simulink model "fec_ber_hw_V2"  (R2020b)
settings: Solver=FixedStepDiscrete  StartTime=0.0  StopTime=T  RelTol=1e-3
values from neighbouring files (symbols this model uses):
  aximm_awgn_reset = 0    [setup.m]
  aximm_bit_count_reset = 0    [setup.m]
  aximm_bits = n_blocks * k    (= 80)    [setup.m]
  aximm_ctrl_word_dec = 0    [setup.m]
  aximm_ctrl_word_enc = 0    [setup.m]
  aximm_enable = 1    [setup.m]
  aximm_length = k * n_blocks    (= 80)    [setup.m]
  aximm_length_dec = n    (= 160)    [setup.m]
  aximm_length_enc = k    (= 80)    [setup.m]
  aximm_llr_mag_reset = 0    [setup.m]
  aximm_llr_scale = (1/noise_var) * llr_scale    (= 1000)    [setup.m]
  aximm_load_dec = 1    [setup.m]
  aximm_load_enc = 1    [setup.m]
  aximm_noise_std = sqrt(noise_var)    [setup.m]
  aximm_reset = 0    [setup.m]
  d = sqrt(-2*log([0:1/4095:1]))    [setup.m]
  fs = 160e6    (= 160000000)    [setup.m]
  generator_polynomial = '''z^13 + z^12 + z^11 + z^8 + 1'''    [setup.m]
  llr_scale = 7.75/7.75    (= 1)    [setup.m]
libraries: simulink x931, hdlsllib x419, commseqgen3 x52, dspsigops x22, commblkcod2 x3, lib_rfsoc_fec x2
(part 47 of 47)

== stateflow chart fec_ber_hw_V2/Encoder Ctrl/Chart ==
  settings: executeAtInitialization=1
  state INIT
    % Local
    count = fi(0,0,32,0);
    n = fi(0,0,32,0);
    loaded_n = fi(0,0,32,0);
    loaded_ctrl = fi(0,0,32,0);
    %
    % DATA Stream
    m_axis_tvalid = false;
    m_axis_tdata = fi(0,0,32,0);
    %
    % CTRL Stream
    m_axis_ctrl_tdata = fi(0,0,32,0);
    m_axis_ctrl_tlast = false;
    m_axis_ctrl_tvalid = false;
    %
    % STATUS Stream
    s_axis_status_tready = false;
  state IDLE
    % Local
    %
    % DATA Stream
    m_axis_tvalid(:) = false;
    m_axis_tdata(:) = 0;
    %
    % CTRL Stream
    m_axis_ctrl_tdata = fi(0,0,32,0);
    m_axis_ctrl_tlast = false;
    m_axis_ctrl_tvalid = false;
    %
    % STATUS Stream
    s_axis_status_tready = false;
  state LOAD_NVALID
    % Local
    loaded_n(:) = block_length;
    loaded_ctrl(:) = ctrl_word;
    %
    % DATA Stream
    m_axis_tvalid(:) = false;
    m_axis_tdata(:) = 0;
    %
    % CTRL Stream
    m_axis_ctrl_tdata(:) = 0;
    m_axis_ctrl_tlast(:) = false;
    m_axis_ctrl_tvalid(:) = false;
    %
    % STATUS Stream
    s_axis_status_tready(:) = true;
  state LOAD_VALID
    % Local
    count(:) = count + 1;
    loaded_n(:) = block_length;
    loaded_ctrl(:) = ctrl_word;
    %
    % DATA Stream
    m_axis_tvalid(:) = true;
    m_axis_tdata(:) = s_axis_tdata;
    %
    % CTRL Stream
    m_axis_ctrl_tdata(:) = 0;
    m_axis_ctrl_tlast(:) = false;
    m_axis_ctrl_tvalid(:) = false;
    %
    % STATUS Stream
    s_axis_status_tready(:) = true;
  state COUNT_DIN
    % Local
    count(:) = count + 1;
    %
    % DATA Stream
    m_axis_tvalid(:) = true;
    m_axis_tdata(:) = s_axis_tdata;       % Complete a full block
    %
    % CTRL Stream
    m_axis_ctrl_tdata(:) = 0;
    m_axis_ctrl_tlast(:) = false;
    m_axis_ctrl_tvalid(:) = false;
    %
    % STATUS Stream
    s_axis_status_tready(:) = true;
  state CTRL
    % Local
    count(:) = count + 1;
    n(:) = loaded_n;
    %
    % DATA Stream
    m_axis_tvalid(:) = true;
    m_axis_tdata(:) = s_axis_tdata;
    %
    % CTRL Stream
    m_axis_ctrl_tdata(:) = loaded_ctrl;
    m_axis_ctrl_tlast(:) = true;
    m_axis_ctrl_tvalid(:) = true;
    %
    % STATUS Stream
    s_axis_status_tready(:) = true;
  state WAITING
    % Local
    %
    % DATA Stream
    m_axis_tvalid(:) = false;
    m_axis_tdata(:) = s_axis_tdata;
    %
    % CTRL Stream
    m_axis_ctrl_tdata(:) = 0;
    m_axis_ctrl_tlast(:) = false;
    m_axis_ctrl_tvalid(:) = false;
    %
    % STATUS Stream
    s_axis_status_tready(:) = true;
  LOAD_VALID -> IDLE [order 3] : [count >= n && s_axis_tvalid == 0]{count(:) = 0}
  (default) -> INIT
  LOAD_NVALID -> COUNT_DIN [order 2] : [s_axis_tvalid == 1 && count > 0]
  LOAD_VALID -> CTRL [order 2] : [count >= n && s_axis_tvalid == 1]{count(:) = 0}
  IDLE -> LOAD_NVALID [order 1] : [load == 1]
  INIT -> IDLE
  LOAD_VALID -> COUNT_DIN [order 1] : [count < n]
  CTRL -> LOAD_VALID [order 1] : [load == 1 && s_axis_tvalid == 1]
  COUNT_DIN -> LOAD_NVALID [order 5] : [load == 1 && s_axis_tvalid == 0]
  LOAD_NVALID -> CTRL [order 1] : [s_axis_tvalid == 1 && count ==0]
  COUNT_DIN -> IDLE [order 3] : [count >= n && s_axis_tvalid == 0]{count(:) = 0}
  IDLE -> CTRL [order 2] : [s_axis_tvalid == 1 && count ==0]
  COUNT_DIN -> LOAD_VALID [order 2] : [load == 1 && s_axis_tvalid == 1]
  COUNT_DIN -> WAITING [order 4] : [load == 0 && s_axis_tvalid == 0]
  CTRL -> COUNT_DIN [order 2] : [s_axis_tvalid == 1]
  COUNT_DIN -> CTRL [order 1] : [count >= n && s_axis_tvalid == 1]{count(:) = 0}
  WAITING -> COUNT_DIN : [s_axis_tvalid == 1]
  CTRL -> WAITING [order 3] : [s_axis_tvalid == 0]
  data: m_axis_ctrl_tvalid output; ctrl_word input; count local; m_axis_ctrl_tdata output; m_axis_ctrl_tlast output; m_axis_tvalid output; block_length input; load input; s_axis_tvalid input; s_axis_status_tready output; n local; loaded_ctrl local; loaded_n local; state output Enum: stateType; s_axis_tdata input; m_axis_tdata output

== matlab function fec_ber_hw_V2/Soft Demodulation/SSR Soft Demodulation Lane 2/Soft Demodulation 10/symmetric_saturation ==
  data: u input; y output
function y = symmetric_saturation(u)
    if u > 7.75
        y = fi(7.75, 1, 6, 2);
    elseif u < -7.75
        y = fi(-7.75, 1, 6, 2);
    else
        y = fi(u, 1, 6, 2);
    end

== matlab function fec_ber_hw_V2/Soft Demodulation/SSR Soft Demodulation Lane 2/Soft Demodulation 11/symmetric_saturation ==
  data: u input; y output
function y = symmetric_saturation(u)
    if u > 7.75
        y = fi(7.75, 1, 6, 2);
    elseif u < -7.75
        y = fi(-7.75, 1, 6, 2);
    else
        y = fi(u, 1, 6, 2);
    end

== matlab function fec_ber_hw_V2/Soft Demodulation/SSR Soft Demodulation Lane 2/Soft Demodulation 12/symmetric_saturation ==
  data: u input; y output
function y = symmetric_saturation(u)
    if u > 7.75
        y = fi(7.75, 1, 6, 2);
    elseif u < -7.75
        y = fi(-7.75, 1, 6, 2);
    else
        y = fi(u, 1, 6, 2);
    end

== matlab function fec_ber_hw_V2/Soft Demodulation/SSR Soft Demodulation Lane 2/Soft Demodulation 13/symmetric_saturation ==
  data: u input; y output
function y = symmetric_saturation(u)
    if u > 7.75
        y = fi(7.75, 1, 6, 2);
    elseif u < -7.75
        y = fi(-7.75, 1, 6, 2);
    else
        y = fi(u, 1, 6, 2);
    end

== matlab function fec_ber_hw_V2/Soft Demodulation/SSR Soft Demodulation Lane 2/Soft Demodulation 14/symmetric_saturation ==
  data: u input; y output
function y = symmetric_saturation(u)
    if u > 7.75
        y = fi(7.75, 1, 6, 2);
    elseif u < -7.75
        y = fi(-7.75, 1, 6, 2);
    else
        y = fi(u, 1, 6, 2);
    end

== matlab function fec_ber_hw_V2/Soft Demodulation/SSR Soft Demodulation Lane 2/Soft Demodulation 15/symmetric_saturation ==
  data: u input; y output
function y = symmetric_saturation(u)
    if u > 7.75
        y = fi(7.75, 1, 6, 2);
    elseif u < -7.75
        y = fi(-7.75, 1, 6, 2);
    else
        y = fi(u, 1, 6, 2);
    end

== matlab function fec_ber_hw_V2/Soft Demodulation/SSR Soft Demodulation Lane 3/Soft Demodulation 1/symmetric_saturation ==
  data: u input; y output
function y = symmetric_saturation(u)
    if u > 7.75
        y = fi(7.75, 1, 6, 2);
    elseif u < -7.75
        y = fi(-7.75, 1, 6, 2);
    else
        y = fi(u, 1, 6, 2);
    end

== matlab function fec_ber_hw_V2/Soft Demodulation/SSR Soft Demodulation Lane 3/Soft Demodulation 2/symmetric_saturation ==
  data: u input; y output
function y = symmetric_saturation(u)
    if u > 7.75
        y = fi(7.75, 1, 6, 2);
    elseif u < -7.75
        y = fi(-7.75, 1, 6, 2);
    else
        y = fi(u, 1, 6, 2);
    end

== matlab function fec_ber_hw_V2/Soft Demodulation/SSR Soft Demodulation Lane 3/Soft Demodulation 3/symmetric_saturation ==
  data: u input; y output
function y = symmetric_saturation(u)
    if u > 7.75
        y = fi(7.75, 1, 6, 2);
    elseif u < -7.75
        y = fi(-7.75, 1, 6, 2);
    else
        y = fi(u, 1, 6, 2);
    end

== matlab function fec_ber_hw_V2/Soft Demodulation/SSR Soft Demodulation Lane 3/Soft Demodulation 4/symmetric_saturation ==
  data: u input; y output
function y = symmetric_saturation(u)
    if u > 7.75
        y = fi(7.75, 1, 6, 2);
    elseif u < -7.75
        y = fi(-7.75, 1, 6, 2);
    else
        y = fi(u, 1, 6, 2);
    end

== matlab function fec_ber_hw_V2/Soft Demodulation/SSR Soft Demodulation Lane 3/Soft Demodulation 5/symmetric_saturation ==
  data: u input; y output
function y = symmetric_saturation(u)
    if u > 7.75
        y = fi(7.75, 1, 6, 2);
    elseif u < -7.75
        y = fi(-7.75, 1, 6, 2);
    else
        y = fi(u, 1, 6, 2);
    end

== matlab function fec_ber_hw_V2/Soft Demodulation/SSR Soft Demodulation Lane 3/Soft Demodulation 6/symmetric_saturation ==
  data: u input; y output
function y = symmetric_saturation(u)
    if u > 7.75
        y = fi(7.75, 1, 6, 2);
    elseif u < -7.75
        y = fi(-7.75, 1, 6, 2);
    else
        y = fi(u, 1, 6, 2);
    end

== matlab function fec_ber_hw_V2/Soft Demodulation/SSR Soft Demodulation Lane 3/Soft Demodulation 7/symmetric_saturation ==
  data: u input; y output
function y = symmetric_saturation(u)
    if u > 7.75
        y = fi(7.75, 1, 6, 2);
    elseif u < -7.75
        y = fi(-7.75, 1, 6, 2);
    else
        y = fi(u, 1, 6, 2);
    end

== matlab function fec_ber_hw_V2/Soft Demodulation/SSR Soft Demodulation Lane 3/Soft Demodulation 8/symmetric_saturation ==
  data: u input; y output
function y = symmetric_saturation(u)
    if u > 7.75
        y = fi(7.75, 1, 6, 2);
    elseif u < -7.75
        y = fi(-7.75, 1, 6, 2);
    else
        y = fi(u, 1, 6, 2);
    end

== matlab function fec_ber_hw_V2/Soft Demodulation/SSR Soft Demodulation Lane 3/Soft Demodulation 0/symmetric_saturation ==
  data: u input; y output
function y = symmetric_saturation(u)
    if u > 7.75
        y = fi(7.75, 1, 6, 2);
    elseif u < -7.75
        y = fi(-7.75, 1, 6, 2);
    else
        y = fi(u, 1, 6, 2);
    end

== matlab function fec_ber_hw_V2/Soft Demodulation/SSR Soft Demodulation Lane 3/Soft Demodulation 9/symmetric_saturation ==
  data: u input; y output
function y = symmetric_saturation(u)
    if u > 7.75
        y = fi(7.75, 1, 6, 2);
    elseif u < -7.75
        y = fi(-7.75, 1, 6, 2);
    else
        y = fi(u, 1, 6, 2);
    end

== matlab function fec_ber_hw_V2/Soft Demodulation/SSR Soft Demodulation Lane 3/Soft Demodulation 10/symmetric_saturation ==
  data: u input; y output
function y = symmetric_saturation(u)
    if u > 7.75
        y = fi(7.75, 1, 6, 2);
    elseif u < -7.75
        y = fi(-7.75, 1, 6, 2);
    else
        y = fi(u, 1, 6, 2);
    end

== matlab function fec_ber_hw_V2/Soft Demodulation/SSR Soft Demodulation Lane 3/Soft Demodulation 11/symmetric_saturation ==
  data: u input; y output
function y = symmetric_saturation(u)
    if u > 7.75
        y = fi(7.75, 1, 6, 2);
    elseif u < -7.75
        y = fi(-7.75, 1, 6, 2);
    else
        y = fi(u, 1, 6, 2);
    end

== matlab function fec_ber_hw_V2/Soft Demodulation/SSR Soft Demodulation Lane 3/Soft Demodulation 12/symmetric_saturation ==
  data: u input; y output
function y = symmetric_saturation(u)
    if u > 7.75
        y = fi(7.75, 1, 6, 2);
    elseif u < -7.75
        y = fi(-7.75, 1, 6, 2);
    else
        y = fi(u, 1, 6, 2);
    end

== matlab function fec_ber_hw_V2/Soft Demodulation/SSR Soft Demodulation Lane 3/Soft Demodulation 13/symmetric_saturation ==
  data: u input; y output
function y = symmetric_saturation(u)
    if u > 7.75
        y = fi(7.75, 1, 6, 2);
    elseif u < -7.75
        y = fi(-7.75, 1, 6, 2);
    else
        y = fi(u, 1, 6, 2);
    end

== matlab function fec_ber_hw_V2/Soft Demodulation/SSR Soft Demodulation Lane 3/Soft Demodulation 14/symmetric_saturation ==
  data: u input; y output
function y = symmetric_saturation(u)
    if u > 7.75
        y = fi(7.75, 1, 6, 2);
    elseif u < -7.75
        y = fi(-7.75, 1, 6, 2);
    else
        y = fi(u, 1, 6, 2);
    end

== matlab function fec_ber_hw_V2/Soft Demodulation/SSR Soft Demodulation Lane 3/Soft Demodulation 15/symmetric_saturation ==
  data: u input; y output
function y = symmetric_saturation(u)
    if u > 7.75
        y = fi(7.75, 1, 6, 2);
    elseif u < -7.75
        y = fi(-7.75, 1, 6, 2);
    else
        y = fi(u, 1, 6, 2);
    end

== matlab function fec_ber_hw_V2/Soft Demodulation/SSR Soft Demodulation Lane 4/Soft Demodulation 0/symmetric_saturation ==
  data: u input; y output
function y = symmetric_saturation(u)
    if u > 7.75
        y = fi(7.75, 1, 6, 2);
    elseif u < -7.75
        y = fi(-7.75, 1, 6, 2);
    else
        y = fi(u, 1, 6, 2);
    end

== matlab function fec_ber_hw_V2/Soft Demodulation/SSR Soft Demodulation Lane 4/Soft Demodulation 1/symmetric_saturation ==
  data: u input; y output
function y = symmetric_saturation(u)
    if u > 7.75
        y = fi(7.75, 1, 6, 2);
    elseif u < -7.75
        y = fi(-7.75, 1, 6, 2);
    else
        y = fi(u, 1, 6, 2);
    end

== matlab function fec_ber_hw_V2/Soft Demodulation/SSR Soft Demodulation Lane 4/Soft Demodulation 2/symmetric_saturation ==
  data: u input; y output
function y = symmetric_saturation(u)
    if u > 7.75
        y = fi(7.75, 1, 6, 2);
    elseif u < -7.75
        y = fi(-7.75, 1, 6, 2);
    else
        y = fi(u, 1, 6, 2);
    end

== matlab function fec_ber_hw_V2/Soft Demodulation/SSR Soft Demodulation Lane 4/Soft Demodulation 3/symmetric_saturation ==
  data: u input; y output
function y = symmetric_saturation(u)
    if u > 7.75
        y = fi(7.75, 1, 6, 2);
    elseif u < -7.75
        y = fi(-7.75, 1, 6, 2);
    else
        y = fi(u, 1, 6, 2);
    end

== matlab function fec_ber_hw_V2/Soft Demodulation/SSR Soft Demodulation Lane 4/Soft Demodulation 4/symmetric_saturation ==
  data: u input; y output
function y = symmetric_saturation(u)
    if u > 7.75
        y = fi(7.75, 1, 6, 2);
    elseif u < -7.75
        y = fi(-7.75, 1, 6, 2);
    else
        y = fi(u, 1, 6, 2);
    end

== matlab function fec_ber_hw_V2/Soft Demodulation/SSR Soft Demodulation Lane 4/Soft Demodulation 5/symmetric_saturation ==
  data: u input; y output
function y = symmetric_saturation(u)
    if u > 7.75
        y = fi(7.75, 1, 6, 2);
    elseif u < -7.75
        y = fi(-7.75, 1, 6, 2);
    else
        y = fi(u, 1, 6, 2);
    end

== matlab function fec_ber_hw_V2/Soft Demodulation/SSR Soft Demodulation Lane 4/Soft Demodulation 6/symmetric_saturation ==
  data: u input; y output
function y = symmetric_saturation(u)
    if u > 7.75
        y = fi(7.75, 1, 6, 2);
    elseif u < -7.75
        y = fi(-7.75, 1, 6, 2);
    else
        y = fi(u, 1, 6, 2);
    end

== matlab function fec_ber_hw_V2/Soft Demodulation1/MATLAB Function ==
  data: u input; y output; reset input
function y = max_magnitude(u, reset)
    persistent max
    
    if isempty(max)
        max = fi(0, 0, 32, 24);
    end

   if abs(u) > max
       max(:) = abs(u);
   end
   
   if reset
       max(:) = 0;
   end
   
   y = fi(max, 0, 32, 24);
    
end

== matlab function fec_ber_hw_V2/Encoder/MATLAB Function5 ==
  data: bits input; valid input; frame input size=[80, 1]; tvalid output; lane_0 output uint32 size=[1,1]
function [tvalid,lane_0] = fcn(bits, valid, frame)

persistent k buffer w buf_i prev_buffer b 

if isempty(k)
    k = 80;
    w = 32;
    prev_buffer = zeros(1,w*8*2)';
    buffer = zeros(1,w*8*2)';
    buf_i = 1;
    lane_0 = uint32(0);
    b = 0;
end

coder.extrinsic('binaryVectorToDecimal'); 

tvalid = false;
lane_0 = uint32(binaryVectorToDecimal(prev_buffer(1:w)','LSBFirst'));

if valid
    buffer(buf_i:buf_i + k - 1) = frame;
    buf_i = buf_i + k;
end

if buf_i >= bits || buf_i >= w || (b + buf_i - 1 == k)
    tvalid = true;
    lane_0 = uint32(binaryVectorToDecimal(buffer(1:w)','LSBFirst'));
    b = b + w;
    
    prev_buffer = buffer;
    
    temp = buffer(w+1:buf_i);
    buf_i = buf_i - w;
    buffer = zeros(1,w*8*2)';
    buffer(1:buf_i) = temp;
    
    if buf_i < 0
        buf_i = 1;
        b = 0;
    end
end

== matlab function fec_ber_hw_V2/Encoder/MATLAB Function ==
  data: u input; y output
function y = fcn(u)

a = u;
% a(a>=0)=-5;
a(a==0)=-1;

y = a;

== matlab function fec_ber_hw_V2/Decode/MATLAB Function3 ==
  data: valid_out output; bits input; valid input; lane_0 input; frame_out output size=[160,1] [80..80]; lane_1 input; lane_2 input; lane_3 input; lane_4 input; lane_5 input; lane_6 input; lane_7 input
function [valid_out, frame_out] = fcn(bits, valid, lane_0, lane_1, lane_2, lane_3, lane_4, lane_5, lane_6, lane_7)

persistent frame buffer buf_0 buf_1 buf_2 buf_3 buf_4 buf_5 buf_6 buf_7 b_count buf_i frame_i out_flag w n;

if isempty(frame)
    n = 160;
    w = 64;
    buffer = zeros(1,n*8)';
    buf_0 = zeros(1,8);
    buf_1 = zeros(1,8);
    buf_2 = zeros(1,8);
    buf_3 = zeros(1,8);
    buf_4 = zeros(1,8);
    buf_5 = zeros(1,8);
    buf_6 = zeros(1,8);
    buf_7 = zeros(1,8);
    buf_i = 1;
    frame_i= 1;
    b_count = 0;
    out_flag = false;
    frame = zeros(1,n)';
end

nt = numerictype(1,6,2);
coder.extrinsic('binaryVectorToDecimal'); 
coder.extrinsic('decimalToBinaryVector'); 

if valid
    lane0_binary = (decimalToBinaryVector(lane_0,w));
    lane1_binary = (decimalToBinaryVector(lane_1,w));
    lane2_binary = (decimalToBinaryVector(lane_2,w));
    lane3_binary = (decimalToBinaryVector(lane_3,w));
    lane4_binary = (decimalToBinaryVector(lane_4,w));
    lane5_binary = (decimalToBinaryVector(lane_5,w));
    lane6_binary = (decimalToBinaryVector(lane_6,w));
    lane7_binary = (decimalToBinaryVector(lane_7,w));
    for i = 0:7
        v_0 = binaryVectorToDecimal(lane0_binary((i*8)+3:(i*8)+8));
        buf_0(i+1) = reinterpretcast(fi(v_0,0,6,0),nt);
        v_1 = binaryVectorToDecimal(lane1_binary((i*8)+3:(i*8)+8));
        buf_1(i+1) = reinterpretcast(fi(v_1,0,6,0),nt);
        v_2 = binaryVectorToDecimal(lane2_binary((i*8)+3:(i*8)+8));
        buf_2(i+1) = reinterpretcast(fi(v_2,0,6,0),nt);
        v_3 = binaryVectorToDecimal(lane3_binary((i*8)+3:(i*8)+8));
        buf_3(i+1) = reinterpretcast(fi(v_3,0,6,0),nt);
        v_4 = binaryVectorToDecimal(lane4_binary((i*8)+3:(i*8)+8));
        buf_4(i+1) = reinterpretcast(fi(v_4,0,6,0),nt);
        v_5 = binaryVectorToDecimal(lane5_binary((i*8)+3:(i*8)+8));
        buf_5(i+1) = reinterpretcast(fi(v_5,0,6,0),nt);
        v_6 = binaryVectorToDecimal(lane6_binary((i*8)+3:(i*8)+8));
        buf_6(i+1) = reinterpretcast(fi(v_6,0,6,0),nt);
        v_7 = binaryVectorToDecimal(lane7_binary((i*8)+3:(i*8)+8));
        buf_7(i+1) = reinterpretcast(fi(v_7,0,6,0),nt);
    end
    buffer(buf_i:buf_i+63) = [buf_0 buf_1 buf_2 buf_3 buf_4 buf_5 buf_6 buf_7];
    buf_i = buf_i + 64;
end

if buf_i > n
    out_flag = true;
end
valid_out = out_flag;

if out_flag
    frame = buffer(frame_i:frame_i+(n-1));
    b_count = b_count + n;
    frame_i = frame_i + n;
    if (frame_i + n - 1) > buf_i - 1
        out_flag = false;
        buf = buffer(frame_i:buf_i - 1);
        buffer = zeros(1,n*8)';
        buf_i = buf_i-frame_i;
        frame_i = 1;
        buffer(1:buf_i) = buf;
        buf_i = buf_i + 1;
    end
end

frame_out = frame(1:160);

== matlab function fec_ber_hw_V2/Soft Demodulation/SSR Soft Demodulation Lane 4/Soft Demodulation 7/symmetric_saturation ==
  data: u input; y output
function y = symmetric_saturation(u)
    if u > 7.75
        y = fi(7.75, 1, 6, 2);
    elseif u < -7.75
        y = fi(-7.75, 1, 6, 2);
    else
        y = fi(u, 1, 6, 2);
    end

== matlab function fec_ber_hw_V2/Soft Demodulation1/MATLAB Function2 ==
  data: valid input; data_i input; frame_i output; data_q input; frame_q output
function [frame_i, frame_q] = fcn(valid, data_i, data_q)

persistent fixed_i 

if isempty(fixed_i)
    fixed_i = 0;
end

coder.extrinsic('decimalToBinaryVector'); 
coder.extrinsic('binaryVectorToDecimal'); 

dout_i = fi(0,0,3,0);
dout_q = fi(0,0,3,0);
frame_i = fi(zeros(1,16),0,3,0);
frame_q = fi(zeros(1,16),0,3,0);
    
if valid
    data_i_bin = fliplr(decimalToBinaryVector(data_i, 48));
    data_q_bin = fliplr(decimalToBinaryVector(data_q, 48));
    
    for i = 1:16
        data_i_dec = binaryVectorToDecimal(data_i_bin(fixed_i*3+1:fixed_i*3+3),'LSBFirst');
        data_q_dec = binaryVectorToDecimal(data_q_bin(fixed_i*3+1:fixed_i*3+3),'LSBFirst');

        dout_i = fi(data_i_dec, 0, 3, 0);
        dout_q = fi(data_q_dec, 0, 3, 0);
        frame_i(i) = dout_i;
        frame_q(i) = dout_q;
        fixed_i = fixed_i + 1;
    end
end

if fixed_i > 15
    fixed_i = 0;
end

== matlab function fec_ber_hw_V2/Soft Demodulation1/Soft Demodulation 0/symmetric_saturation ==
  data: u input; y output
function y = symmetric_saturation(u)
    if u > 7.75
        y = fi(7.75, 1, 6, 2);
    elseif u < -7.75
        y = fi(-7.75, 1, 6, 2);
    else
        y = fi(u, 1, 6, 2);
    end

== matlab function fec_ber_hw_V2/Soft Demodulation1/MATLAB Function1 ==
  data: valid input; data_i input; dout_i output; data_q input; dout_q output
function [dout_i, dout_q] = fcn(valid, data_i, data_q)

persistent fixed_i 

if isempty(fixed_i)
    fixed_i = 0;
end

coder.extrinsic('decimalToBinaryVector'); 
coder.extrinsic('binaryVectorToDecimal'); 

dout_i = fi(0,0,3,0);
dout_q = fi(0,0,3,0);
if valid
    data_i_bin = fliplr(decimalToBinaryVector(data_i, 48));
    data_q_bin = fliplr(decimalToBinaryVector(data_q, 48));
    
    data_i_dec = binaryVectorToDecimal(data_i_bin(fixed_i*3+1:fixed_i*3+3),'LSBFirst');
    data_q_dec = binaryVectorToDecimal(data_q_bin(fixed_i*3+1:fixed_i*3+3),'LSBFirst');
    
    dout_i = fi(data_i_dec, 0, 3, 0);
    dout_q = fi(data_q_dec, 0, 3, 0);
    fixed_i = fixed_i + 1;
end

if fixed_i > 15
    fixed_i = 0;
end

== matlab function fec_ber_hw_V2/Encoder/MATLAB Function4 ==
  data: bits input; valid input; frame input size=[160, 1]; tvalid output; lane_0 output size=[1,1]
function [tvalid,lane_0] = fcn(bits, valid, frame)

persistent n buffer w buf_i prev_buffer b 

if isempty(n)
    n = 160;
    w = 64;
    b = 0;
    prev_buffer = false(1,w*8*4)';
    buffer = false(1,w*8*4)';
    buf_i = 1;
    lane_0 = uint64(0);
end

coder.extrinsic('binaryVectorToDecimal'); 

tvalid = false;
lane_0 = binaryVectorToDecimal(prev_buffer(1:64)','LSBFirst');

if valid
    buffer(buf_i:buf_i + n - 1) = frame;
    buf_i = buf_i + n;
    b = b + 160;
end

if ((b > 0) || (buf_i >= w))
       
    tvalid = true;
    lane_0 = binaryVectorToDecimal(buffer(1:64)','LSBFirst');
    b = b - 64;
    prev_buffer = buffer;
    
    temp = buffer(64+1:buf_i);
    buf_i = buf_i - 64;
    buffer = false(1,w*8*4)';
    buffer(1:buf_i) = temp;
end

== matlab function fec_ber_hw_V2/Encoder/MATLAB Function3 ==
  data: valid_out output; bits input; valid input; lane_0 input; frame_out output size=[80,1] [80..80]
function [valid_out, frame_out] = fcn(bits, valid, lane_0)

persistent frame fixed_frame frame_i fixed_i k w out_flag bit_count

if isempty(frame)
    k = 80;
    w = 32;
    frame = zeros(1,k)';
    fixed_frame = zeros(1,w*32)';
    frame_i = 1;
    fixed_i = 1;
    out_flag = false;
    bit_count = 0;
end

coder.extrinsic('decimalToBinaryVector');

if valid
    fixed_frame(fixed_i:fixed_i+w) = fliplr(decimalToBinaryVector(lane_0,w));
    fixed_i = fixed_i + w;
end

if fixed_i >= k
    out_flag = true;
end

valid_out = out_flag;

if out_flag
    frame = fixed_frame(frame_i:frame_i+(k-1));
    bit_count = bit_count + k;
    frame_i = frame_i + k;
    if (frame_i + k - 1) > fixed_i - 1
        out_flag = false;
        buf = fixed_frame(frame_i:fixed_i - 1);
        fixed_frame = zeros(1,w*32)';
        fixed_i = fixed_i-frame_i;
        frame_i = 1;
        fixed_frame(1:fixed_i) = buf;
        fixed_i = fixed_i + 1;
    end
end

if (bit_count > bits)
    valid_out = false;
end

frame_out = frame(1:80);

== matlab function fec_ber_hw_V2/Decode/MATLAB Function5 ==
  data: bits input; valid input; frame input size=[80, 1]; tvalid output; lane_0 output uint32 size=[1,1]
function [tvalid,lane_0] = fcn(bits, valid, frame)

persistent k buffer w buf_i prev_buffer b 

if isempty(k)
    k = 80;
    w = 32;
    prev_buffer = zeros(1,w*8*2)';
    buffer = zeros(1,w*8*2)';
    buf_i = 1;
    lane_0 = uint32(0);
    b = 0;
end

coder.extrinsic('binaryVectorToDecimal'); 

tvalid = false;
lane_0 = uint32(binaryVectorToDecimal(prev_buffer(1:w)','LSBFirst'));

if valid
    buffer(buf_i:buf_i + k - 1) = frame;
    buf_i = buf_i + k;
end

if buf_i >= bits || buf_i >= w || (b + buf_i - 1 == k)
    tvalid = true;
    lane_0 = uint32(binaryVectorToDecimal(buffer(1:w)','LSBFirst'));
    b = b + w;
    
    prev_buffer = buffer;
    
    temp = buffer(w+1:buf_i);
    buf_i = buf_i - w;
    buffer = zeros(1,w*8*2)';
    buffer(1:buf_i) = temp;
    
    if buf_i < 0
        buf_i = 1;
        b = 0;
    end
end
